simulink model "impendent_control"  (R2020b)
settings: Solver=FixedStepAuto  StartTime=0  StopTime=20  FixedStep=0.002  RelTol=1e-3
settings Model: Creator=lsk  LastModifiedBy=lsk

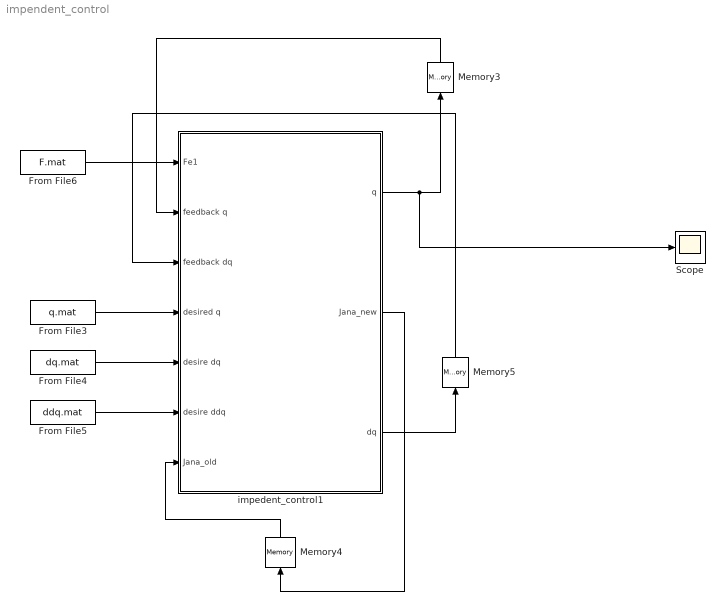
== system impendent_control ==
  From File3 : FromFile  FileName=q.mat
  From File4 : FromFile  FileName=dq.mat
  From File5 : FromFile  FileName=ddq.mat
  From File6 : FromFile  FileName=F.mat
  Memory3 : Memory  InitialCondition="[-1.26423369443190\t-1.44424631137251\t1.62606583856285\t-1.18060848187035\t-1.67197070062840\t-1.04318229967319]"
  Memory4 : Memory  InitialCondition="[-0.266147571210034\t-0.0228642277800098\t0.0561694595006700\t0.0432367769486852\t-0.0908701336324438\t0;-0.185625730629766\t0.0722313558368560\t-0.177447331936746\t-0.136591143644473\t-0.0343556248257271\t0;0\t-0.309757599949874\t-0.276437498712455\t-0.0433441320109634\t-0.00828008794975587\t0;0\t-0.611286356998400\t-0.611286356998400\t-0.611286356998400\t0.773691656626561\t-0.433817753420009;0\t0.832951080784977\t0.832951080784977\t0.832951080784977\t0.465262723808915\t-0.382135972757221;1\t-0.259766266542128\t-0.259766266542128\t-0.259766266542128\t-0.212540535977552\t-1.02086724969865]"
  Memory5 : Memory  InitialCondition="[0.0749188626195236\t0.110703858237117\t-0.193787178596464\t0.0894245369746680\t0.0405634935859376\t0.0633059717930151]"
  Scope : Scope
  impedent_control1 : Subsystem  mask{m_M=[1 1 1 1 1 1]*0.2, m_B=[1 1 1 1 1 1]*5, m_K=[1 1 1 1 1 1]*3}
      mask prompts: m_M "M"; m_B "B"; m_K "K"
  wires:
  From File6/1 -> impedent_control1/1(Fe1)
  From File4/1 -> impedent_control1/5(desire dq)
  impedent_control1/3(dq) -> Memory5/1
  Memory5/1 -> impedent_control1/3(feedback dq)
  impedent_control1/1(q) -> Scope/1, Memory3/1
  Memory3/1 -> impedent_control1/2(feedback q)
  Memory4/1 -> impedent_control1/7("Jana_old ")
  From File5/1 -> impedent_control1/6(desire ddq)
  impedent_control1/2(Jana_new) -> Memory4/1
  From File3/1 -> impedent_control1/4(desired q)

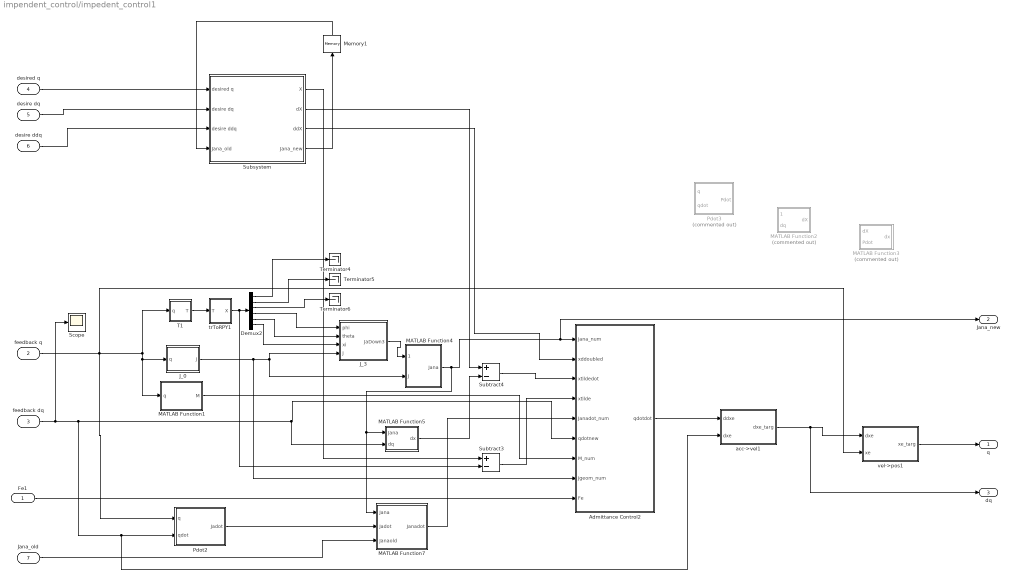
== system impendent_control/impedent_control1 ==
  Fe1 : Inport
  feedback q : Inport  Port=2
  feedback dq : Inport  Port=3
  desired q : Inport  Port=4
  desire dq : Inport  Port=5
  desire ddq : Inport  Port=6
  "Jana_old " : Inport  Port=7
  Admittance Control2 : MATLAB Function  TreatAsAtomicUnit=on
  Demux2 : Demux  Outputs=6
  J_0 : MATLAB Function  TreatAsAtomicUnit=on
  J_3 : MATLAB Function  TreatAsAtomicUnit=on
  MATLAB Function1 : MATLAB Function  TreatAsAtomicUnit=on
  MATLAB Function2 : MATLAB Function  Commented=on  TreatAsAtomicUnit=on
  MATLAB Function3 : MATLAB Function  Commented=on  TreatAsAtomicUnit=on
  MATLAB Function4 : MATLAB Function  TreatAsAtomicUnit=on
  MATLAB Function5 : MATLAB Function  TreatAsAtomicUnit=on
  MATLAB Function7 : MATLAB Function  TreatAsAtomicUnit=on
  Memory1 : Memory  InitialCondition="[-0.266147571210034\t-0.0228642277800098\t0.0561694595006700\t0.0432367769486852\t-0.0908701336324438\t0;-0.185625730629766\t0.0722313558368560\t-0.177447331936746\t-0.136591143644473\t-0.0343556248257271\t0;0\t-0.309757599949874\t-0.276437498712455\t-0.0433441320109634\t-0.00828008794975587\t0;0\t-0.611286356998400\t-0.611286356998400\t-0.611286356998400\t0.773691656626561\t-0.433817753420009;0\t0.832951080784977\t0.832951080784977\t0.832951080784977\t0.465262723808915\t-0.382135972757221;1\t-0.259766266542128\t-0.259766266542128\t-0.259766266542128\t-0.212540535977552\t-1.02086724969865]"
  Pdot2 : MATLAB Function  TreatAsAtomicUnit=on
  Pdot3 : MATLAB Function  Commented=on  TreatAsAtomicUnit=on
  Scope : Scope
  Subsystem : Subsystem
  Subtract3 : Sum  Inputs=+-
  Subtract4 : Sum  Inputs=+-
  T1 : MATLAB Function  TreatAsAtomicUnit=on
  Terminator4 : Terminator
  Terminator5 : Terminator
  Terminator6 : Terminator
  acc->vel1 : MATLAB Function  TreatAsAtomicUnit=on
  trToRPY1 : MATLAB Function  TreatAsAtomicUnit=on
  vel->pos1 : MATLAB Function  TreatAsAtomicUnit=on
  q : Outport
  Jana_new : Outport  Port=2
  dq : Outport  Port=3
  wires:
  acc->vel1/1(dxe_targ) -> dq/1, vel->pos1/1(dxe)
  T1/1(T) -> trToRPY1/1(T)
  trToRPY1/1(X) -> Subtract3/2, Demux2/1
  Demux2/3 -> Terminator6/1
  Demux2/2 -> Terminator5/1
  Demux2/1 -> Terminator4/1
  vel->pos1/1(xe_targ) -> q/1
  desired q/1 -> Subsystem/1(desired q)
  desire dq/1 -> Subsystem/2(desire dq)
  desire ddq/1 -> Subsystem/3(desire ddq)
  Subsystem/4(Jana_new) -> Memory1/1
  Memory1/1 -> Subsystem/4(Jana_old)
  feedback q/1 -> vel->pos1/2(xe), Pdot2/1(q), J_0/1(q), MATLAB Function1/1(q), T1/1(q)
  Demux2/4 -> J_3/1(phi)
  Demux2/5 -> J_3/2(theta)
  Demux2/6 -> J_3/3(xi)
  J_0/1(J) -> Admittance Control2/8(Jgeom_num), MATLAB Function4/2(J), J_3/4(J)
  J_3/1(JaDown3) -> MATLAB Function4/1(JaDown3)
  Subsystem/3(ddX) -> Admittance Control2/2(xddoubled)
  MATLAB Function4/1(Jana) -> MATLAB Function5/1(Jana), MATLAB Function7/1(Jana), Jana_new/1, Admittance Control2/1(Jana_num)
  feedback dq/1 -> acc->vel1/2(dxe), Pdot2/2(qdot), MATLAB Function5/2(dq), Admittance Control2/6(qdotnew), Scope/1
  Subsystem/2(dX) -> Subtract4/1
  MATLAB Function1/1(M) -> Admittance Control2/7(M_num)
  MATLAB Function5/1(dx) -> Subtract4/2
  Subtract4/1 -> Admittance Control2/3(xtildedot)
  Subsystem/1(X) -> Subtract3/1
  Subtract3/1 -> Admittance Control2/4(xtilde)
  Fe1/1 -> Admittance Control2/9(Fe)
  "Jana_old "/1 -> MATLAB Function7/3(Janaold)
  Pdot2/1(Jadot) -> MATLAB Function7/2(Jadot)
  MATLAB Function7/1(Janadot) -> Admittance Control2/5(Janadot_num)
  Admittance Control2/1(qdotdot) -> acc->vel1/1(ddxe)

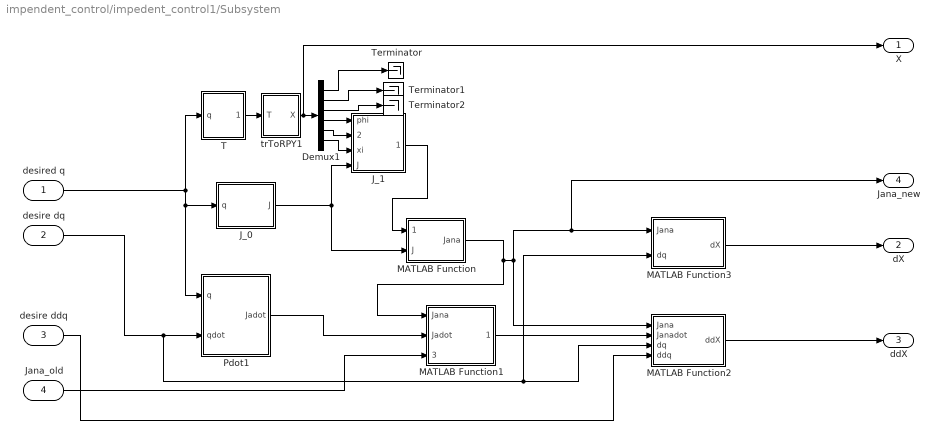
== system impendent_control/impedent_control1/Subsystem ==
  desired q : Inport
  desire dq : Inport  Port=2
  desire ddq : Inport  Port=3
  Jana_old : Inport  Port=4
  Demux1 : Demux  Outputs=6
  J_0 : MATLAB Function  TreatAsAtomicUnit=on
  J_1 : MATLAB Function  TreatAsAtomicUnit=on
  MATLAB Function : MATLAB Function  TreatAsAtomicUnit=on
  MATLAB Function1 : MATLAB Function  TreatAsAtomicUnit=on
  MATLAB Function2 : MATLAB Function  TreatAsAtomicUnit=on
  MATLAB Function3 : MATLAB Function  TreatAsAtomicUnit=on
  Pdot1 : MATLAB Function  TreatAsAtomicUnit=on
  T : MATLAB Function  TreatAsAtomicUnit=on
  Terminator : Terminator
  Terminator1 : Terminator
  Terminator2 : Terminator
  trToRPY1 : MATLAB Function  TreatAsAtomicUnit=on
  X : Outport
  dX : Outport  Port=2
  ddX : Outport  Port=3
  Jana_new : Outport  Port=4
  wires:
  desired q/1 -> Pdot1/1(q), J_0/1(q), T/1(q)
  T/1(T_fin) -> trToRPY1/1(T)
  Demux1/1 -> Terminator/1
  Demux1/2 -> Terminator1/1
  Demux1/6 -> J_1/3(xi)
  Demux1/3 -> Terminator2/1
  Demux1/4 -> J_1/1(phi)
  Demux1/5 -> J_1/2(theta)
  trToRPY1/1(X) -> X/1, Demux1/1
  J_0/1(J) -> MATLAB Function/2(J), J_1/4(J)
  J_1/1(JaDown3) -> MATLAB Function/1(JaDown3)
  desire dq/1 -> MATLAB Function2/3(dq), MATLAB Function3/2(dq), Pdot1/2(qdot)
  MATLAB Function/1(Jana) -> MATLAB Function1/1(Jana), MATLAB Function2/1(Jana), Jana_new/1, MATLAB Function3/1(Jana)
  Pdot1/1(Jadot) -> MATLAB Function1/2(Jadot)
  Jana_old/1 -> MATLAB Function1/3(Janaold)
  MATLAB Function3/1(dX) -> dX/1
  MATLAB Function1/1(Janadot) -> MATLAB Function2/2(Janadot)
  desire ddq/1 -> MATLAB Function2/4(ddq)
  MATLAB Function2/1(ddX) -> ddX/1

== matlab function impendent_control/impedent_control1/MATLAB Function7 ==
  data: Jana input; Jadot input; Janadot output; Janaold input
function Janadot = fcn(Jana,Jadot,Janaold)
Jadown3 = Jana - Janaold;
Janadot=[Jadot(1:3,:);Jadown3(4:6,:)];
end

== matlab function impendent_control/impedent_control1/Pdot2 ==
  data: q input; qdot input; Jadot output
function Jadot = Jadot(q,qdot)
%JADOT
%    JADOT = JADOT(Q1,Q2,Q3,Q4,Q5,Q1DOT,Q2DOT,Q3DOT,Q4DOT,Q5DOT)

%    This function was generated by the Symbolic Math Toolbox version 8.6.
%    07-Dec-2021 14:58:16
q1=q(1);q2=q(2);q3=q(3);q4=q(4);q5=q(5);q6=q(6);
q1dot=qdot(1);q2dot=qdot(2);q3dot=qdot(3);q4dot=qdot(4);q5dot=qdot(5);q6dot=qdot(6);
t2 = cos(q1);
t3 = cos(q2);
t4 = cos(q3);
t5 = cos(q4);
t6 = cos(q5);
t7 = sin(q1);
t8 = sin(q2);
t9 = sin(q3);
t10 = sin(q4);
t11 = sin(q5);
t12 = q2+q3+q4;
t13 = q2dot+q3dot+q4dot;
t14 = cos(t12);
t15 = sin(t12);
t16 = t6.*(3.9e+1./4.0e+2);
t17 = t5.*(5.7e+1./5.0e+2);
t18 = t10.*(5.7e+1./5.0e+2);
t22 = t5.*t11.*(3.9e+1./4.0e+2);
t23 = t10.*t11.*(3.9e+1./4.0e+2);
t24 = q4dot.*t10.*(-5.7e+1./5.0e+2);
t30 = q5dot.*t5.*t6.*(-3.9e+1./4.0e+2);
t19 = -t18;
t20 = q4dot.*t17;
t21 = q4dot.*t18;
t25 = -t22;
t26 = q5dot.*t5.*t16;
t27 = q4dot.*t22;
t28 = q5dot.*t10.*t16;
t29 = q4dot.*t23;
t31 = t16+1.065e-1;
t32 = t17+t23;
t33 = t18+t25;
t34 = t4.*t32;
t35 = t9.*t32;
t46 = t19+t22+2.37e+2./1.0e+3;
t51 = t20+t29+t30;
t52 = t24+t27+t28;
t36 = q3dot.*t34;
t37 = q3dot.*t35;
t38 = t4.*t33;
t39 = t9.*t33;
t42 = -t35;
t47 = t4.*t46;
t48 = t9.*t46;
t53 = t4.*t51;
t54 = t4.*t52;
t55 = t9.*t51;
t56 = t9.*t52;
t40 = q3dot.*t38;
t41 = q3dot.*t39;
t43 = -t37;
t44 = -t39;
t49 = q3dot.*t47;
t50 = q3dot.*t48;
t57 = -t54;
t58 = -t55;
t59 = t35+t38;
t66 = t34+t48;
t67 = t42+t47;
t72 = -t8.*(t35-t47);
t75 = -q2dot.*t3.*(t35-t47);
t45 = -t41;
t60 = t34+t44;
t61 = t8.*t59;
t62 = q2dot.*t3.*t59;
t68 = t3.*t66;
t69 = t8.*t66;
t76 = t67+3.3e+1./1.25e+2;
t85 = t37+t40+t55+t57;
t89 = t36+t50+t53+t56;
t92 = t43+t49+t54+t58;
t94 = -t3.*(t37-t49+t55+t57);
t95 = -t8.*(t37-t49+t55+t57);
t63 = t3.*t60;
t64 = -t61;
t65 = q2dot.*t8.*t60;
t70 = q2dot.*t69;
t71 = q2dot.*t68;
t73 = -t69;
t77 = t3.*t76;
t78 = t8.*t76;
t82 = t68+t72;
t84 = t36+t45+t53+t56;
t87 = t3.*t85;
t90 = t3.*t89;
t91 = t8.*t89;
t74 = -t70;
t79 = q2dot.*t78;
t80 = q2dot.*t77;
t81 = t63+t64;
t83 = t68+t78;
t86 = t73+t77;
t88 = t8.*t84;
t93 = -t91;
t96 = t62+t65+t87+t88;
t97 = t74+t75+t93+t94;
t98 = t71+t79+t90+t95;
t99 = t74+t80+t93+t94;
Jadot = reshape([-t7.*t98-q5dot.*t2.*t11.*(3.9e+1./4.0e+2)-q1dot.*t7.*t31-q1dot.*t2.*(t69-t77),t2.*t98-q5dot.*t7.*t11.*(3.9e+1./4.0e+2)+q1dot.*t2.*t31-q1dot.*t7.*(t69-t77),0.0,-t2.*(t70-t80+t91+t3.*(t37-t49+t55+t57))-q1dot.*t7.*t83,-t7.*(t70-t80+t91+t3.*(t37-t49+t55+t57))+q1dot.*t2.*t83,t98,-t2.*(t70+t91+t3.*(t37-t49+t55+t57)+q2dot.*t3.*(t35-t47))-q1dot.*t7.*t82,-t7.*(t70+t91+t3.*(t37-t49+t55+t57)+q2dot.*t3.*(t35-t47))+q1dot.*t2.*t82,t71+t90+t95+q2dot.*t72,-t2.*t96+q1dot.*t7.*(t61-t63),-t7.*t96-q1dot.*t2.*(t61-t63),q2dot.*t63+q2dot.*t64+t3.*t84-t8.*t85,q1dot.*t2.*t11.*(-3.9e+1./4.0e+2)-q5dot.*t6.*t7.*(3.9e+1./4.0e+2)+q5dot.*t2.*t11.*t14.*(3.9e+1./4.0e+2)+q1dot.*t7.*t14.*t16+t2.*t13.*t15.*t16,q1dot.*t7.*t11.*(-3.9e+1./4.0e+2)+q5dot.*t2.*t16-q1dot.*t2.*t6.*t14.*(3.9e+1./4.0e+2)+q5dot.*t7.*t11.*t14.*(3.9e+1./4.0e+2)+t7.*t13.*t15.*t16,q5dot.*t11.*t15.*(3.9e+1./4.0e+2)-t6.*t13.*t14.*(3.9e+1./4.0e+2),0.0,0.0,0.0],[3,6]);

end

== matlab function impendent_control/impedent_control1/Pdot3 ==
  data: q input; qdot input; Pdot output
% function Pdot = Pdot(q1,q2,q3,q4,q5,q1dot,q2dot,q3dot,q4dot,q5dot)
function Pdot = Pdot(q,qdot)
q1=q(1);q2=q(2);q3=q(3);q4=q(4);q5=q(5);q6=q(6);
q1dot=qdot(1);q2dot=qdot(2);q3dot=qdot(3);q4dot=qdot(4);q5dot=qdot(5);q6dot=qdot(6);
%PDOT
%    PDOT = PDOT(Q1,Q2,Q3,Q4,Q5,Q1DOT,Q2DOT,Q3DOT,Q4DOT,Q5DOT)

%    This function was generated by the Symbolic Math Toolbox version 8.6.
%    07-Dec-2021 16:11:39

t2 = cos(q1);
t3 = cos(q2);
t4 = cos(q3);
t5 = cos(q4);
t6 = cos(q5);
t7 = sin(q1);
t8 = sin(q2);
t9 = sin(q3);
t10 = sin(q4);
t11 = sin(q5);
t12 = t6.*(3.9e+1./4.0e+2);
t13 = t5.*(5.7e+1./5.0e+2);
t14 = t10.*(5.7e+1./5.0e+2);
t18 = t5.*t11.*(3.9e+1./4.0e+2);
t19 = t10.*t11.*(3.9e+1./4.0e+2);
t20 = q4dot.*t10.*(-5.7e+1./5.0e+2);
t25 = q5dot.*t5.*t6.*(-3.9e+1./4.0e+2);
t15 = -t14;
t16 = q4dot.*t13;
t17 = q4dot.*t14;
t21 = q5dot.*t5.*t12;
t22 = q4dot.*t18;
t23 = q5dot.*t10.*t12;
t24 = q4dot.*t19;
t26 = t12+1.065e-1;
t27 = t13+t19;
t28 = t4.*t27;
t29 = t9.*t27;
t34 = t15+t18+2.37e+2./1.0e+3;
t39 = t16+t24+t25;
t40 = t20+t22+t23;
t30 = q3dot.*t28;
t31 = q3dot.*t29;
t32 = -t29;
t35 = t4.*t34;
t36 = t9.*t34;
t41 = t4.*t39;
t42 = t4.*t40;
t43 = t9.*t39;
t44 = t9.*t40;
t33 = -t31;
t37 = q3dot.*t35;
t38 = q3dot.*t36;
t45 = -t43;
t46 = t28+t36;
t50 = t32+t35+3.3e+1./1.25e+2;
t47 = t8.*t46;
t48 = q2dot.*t3.*t46;
t51 = t3.*t50;
t52 = q2dot.*t8.*t50;
t54 = t30+t38+t41+t44;
t56 = t33+t37+t42+t45;
t57 = -t8.*(t31-t37-t42+t43);
t49 = -t47;
t55 = t3.*t54;
t53 = t49+t51;
t58 = t48+t52+t55+t57;
Pdot = [t2.*t58-q5dot.*t7.*t11.*(3.9e+1./4.0e+2)+q1dot.*t2.*t26-q1dot.*t7.*(t47-t51);t7.*t58+q5dot.*t2.*t11.*(3.9e+1./4.0e+2)+q1dot.*t7.*t26+q1dot.*t2.*(t47-t51);q2dot.*t47-q2dot.*t51+t8.*t54+t3.*(t31-t37-t42+t43)];


end

== matlab function impendent_control/impedent_control1/Subsystem/J_0 ==
  data: q input; J output
function J = J(q)
q1=q(1);q2=q(2);q3=q(3);q4=q(4);q5=q(5);q6=q(6);
%J
%    J = J(Q1,Q2,Q3,Q4,Q5)

%    This function was generated by the Symbolic Math Toolbox version 8.6.
%    07-Dec-2021 11:30:25

t2 = cos(q1);
t3 = cos(q2);
t4 = cos(q3);
t5 = cos(q4);
t6 = cos(q5);
t7 = sin(q1);
t8 = sin(q2);
t9 = sin(q3);
t10 = sin(q4);
t11 = sin(q5);
t12 = q2+q3+q4;
t13 = cos(t12);
t14 = sin(t12);
t15 = -t2;
t16 = t6.*(3.9e+1./4.0e+2);
t17 = t5.*(5.7e+1./5.0e+2);
t18 = t10.*(5.7e+1./5.0e+2);
t20 = t5.*t11.*(3.9e+1./4.0e+2);
t21 = t10.*t11.*(3.9e+1./4.0e+2);
t19 = -t18;
t22 = -t20;
t23 = t16+1.065e-1;
t24 = t17+t21;
t25 = t18+t22;
t26 = t4.*t24;
t27 = t9.*t24;
t32 = t19+t20+2.37e+2./1.0e+3;
t28 = t4.*t25;
t29 = t9.*t25;
t30 = -t27;
t33 = t4.*t32;
t34 = t9.*t32;
t31 = -t29;
t35 = t27+t28;
t40 = t26+t34;
t41 = t30+t33;
t44 = -t8.*(t27-t33);
t36 = t26+t31;
t37 = t8.*t35;
t42 = t3.*t40;
t43 = t8.*t40;
t46 = t41+3.3e+1./1.25e+2;
t38 = t3.*t36;
t39 = -t37;
t45 = -t43;
t47 = t3.*t46;
t48 = t8.*t46;
t50 = t42+t44;
t49 = t38+t39;
t51 = t42+t48;
t52 = t45+t47;
J = reshape([t2.*t23-t7.*(t43-t47),t7.*t23+t2.*(t43-t47),0.0,0.0,0.0,1.0,t2.*t51,t7.*t51,t43-t47,t7,t15,0.0,t2.*t50,t7.*t50,t43+t3.*(t27-t33),t7,t15,0.0,-t2.*(t37-t38),-t7.*(t37-t38),t3.*t35+t8.*t36,t7,t15,0.0,t7.*t11.*(-3.9e+1./4.0e+2)-t2.*t6.*t13.*(3.9e+1./4.0e+2),t2.*t11.*(3.9e+1./4.0e+2)-t6.*t7.*t13.*(3.9e+1./4.0e+2),t6.*t14.*(-3.9e+1./4.0e+2),t2.*t14,t7.*t14,-t13,0.0,0.0,0.0,t6.*t7+t11.*t13.*t15,t6.*t15-t7.*t11.*t13,-t11.*t14],[6,6]);


end

== matlab function impendent_control/impedent_control1/Subsystem/J_1 ==
  data: phi input; JaDown3 output; theta input; xi input; J input
function JaDown3 = Jana(phi,theta,xi,J)
om2eulmat=[cos(theta)*cos(xi), -sin(xi), 0;
    cos(theta)*sin(xi),  cos(xi), 0;
    -sin(theta),       0, 1];
omega=J(4:6,:);
JaDown3 = om2eulmat\omega;
end

== matlab function impendent_control/impedent_control1/Subsystem/MATLAB Function ==
  data: JaDown3 input; Jana output; J input
function Jana = fcn(JaDown3,J)
Jana=[J(1:3,:);JaDown3];
end

== matlab function impendent_control/impedent_control1/Subsystem/MATLAB Function1 ==
  data: Jana input; Jadot input; Janadot output; Janaold input
function Janadot = fcn(Jana,Jadot,Janaold)
Jadown3 = Jana - Janaold;
Janadot=[Jadot(1:3,:);Jadown3(4:6,:)];
end

== matlab function impendent_control/impedent_control1/Subsystem/MATLAB Function2 ==
  data: Jana input; Janadot input; dq input; ddX output; ddq input
function ddX = getddX(Jana,Janadot,dq,ddq)
ddX = Janadot * dq + Jana * ddq;

== matlab function impendent_control/impedent_control1/Subsystem/MATLAB Function3 ==
  data: Jana input; dX output; dq input
function dX = getdX(Jana,dq)
dX=Jana*dq;

== matlab function impendent_control/impedent_control1/Subsystem/Pdot1 ==
  data: q input; qdot input; Jadot output
function Jadot = Jadot(q,qdot)
%JADOT
%    JADOT = JADOT(Q1,Q2,Q3,Q4,Q5,Q1DOT,Q2DOT,Q3DOT,Q4DOT,Q5DOT)

%    This function was generated by the Symbolic Math Toolbox version 8.6.
%    07-Dec-2021 14:58:16
q1=q(1);q2=q(2);q3=q(3);q4=q(4);q5=q(5);q6=q(6);
q1dot=qdot(1);q2dot=qdot(2);q3dot=qdot(3);q4dot=qdot(4);q5dot=qdot(5);q6dot=qdot(6);
t2 = cos(q1);
t3 = cos(q2);
t4 = cos(q3);
t5 = cos(q4);
t6 = cos(q5);
t7 = sin(q1);
t8 = sin(q2);
t9 = sin(q3);
t10 = sin(q4);
t11 = sin(q5);
t12 = q2+q3+q4;
t13 = q2dot+q3dot+q4dot;
t14 = cos(t12);
t15 = sin(t12);
t16 = t6.*(3.9e+1./4.0e+2);
t17 = t5.*(5.7e+1./5.0e+2);
t18 = t10.*(5.7e+1./5.0e+2);
t22 = t5.*t11.*(3.9e+1./4.0e+2);
t23 = t10.*t11.*(3.9e+1./4.0e+2);
t24 = q4dot.*t10.*(-5.7e+1./5.0e+2);
t30 = q5dot.*t5.*t6.*(-3.9e+1./4.0e+2);
t19 = -t18;
t20 = q4dot.*t17;
t21 = q4dot.*t18;
t25 = -t22;
t26 = q5dot.*t5.*t16;
t27 = q4dot.*t22;
t28 = q5dot.*t10.*t16;
t29 = q4dot.*t23;
t31 = t16+1.065e-1;
t32 = t17+t23;
t33 = t18+t25;
t34 = t4.*t32;
t35 = t9.*t32;
t46 = t19+t22+2.37e+2./1.0e+3;
t51 = t20+t29+t30;
t52 = t24+t27+t28;
t36 = q3dot.*t34;
t37 = q3dot.*t35;
t38 = t4.*t33;
t39 = t9.*t33;
t42 = -t35;
t47 = t4.*t46;
t48 = t9.*t46;
t53 = t4.*t51;
t54 = t4.*t52;
t55 = t9.*t51;
t56 = t9.*t52;
t40 = q3dot.*t38;
t41 = q3dot.*t39;
t43 = -t37;
t44 = -t39;
t49 = q3dot.*t47;
t50 = q3dot.*t48;
t57 = -t54;
t58 = -t55;
t59 = t35+t38;
t66 = t34+t48;
t67 = t42+t47;
t72 = -t8.*(t35-t47);
t75 = -q2dot.*t3.*(t35-t47);
t45 = -t41;
t60 = t34+t44;
t61 = t8.*t59;
t62 = q2dot.*t3.*t59;
t68 = t3.*t66;
t69 = t8.*t66;
t76 = t67+3.3e+1./1.25e+2;
t85 = t37+t40+t55+t57;
t89 = t36+t50+t53+t56;
t92 = t43+t49+t54+t58;
t94 = -t3.*(t37-t49+t55+t57);
t95 = -t8.*(t37-t49+t55+t57);
t63 = t3.*t60;
t64 = -t61;
t65 = q2dot.*t8.*t60;
t70 = q2dot.*t69;
t71 = q2dot.*t68;
t73 = -t69;
t77 = t3.*t76;
t78 = t8.*t76;
t82 = t68+t72;
t84 = t36+t45+t53+t56;
t87 = t3.*t85;
t90 = t3.*t89;
t91 = t8.*t89;
t74 = -t70;
t79 = q2dot.*t78;
t80 = q2dot.*t77;
t81 = t63+t64;
t83 = t68+t78;
t86 = t73+t77;
t88 = t8.*t84;
t93 = -t91;
t96 = t62+t65+t87+t88;
t97 = t74+t75+t93+t94;
t98 = t71+t79+t90+t95;
t99 = t74+t80+t93+t94;
Jadot = reshape([-t7.*t98-q5dot.*t2.*t11.*(3.9e+1./4.0e+2)-q1dot.*t7.*t31-q1dot.*t2.*(t69-t77),t2.*t98-q5dot.*t7.*t11.*(3.9e+1./4.0e+2)+q1dot.*t2.*t31-q1dot.*t7.*(t69-t77),0.0,-t2.*(t70-t80+t91+t3.*(t37-t49+t55+t57))-q1dot.*t7.*t83,-t7.*(t70-t80+t91+t3.*(t37-t49+t55+t57))+q1dot.*t2.*t83,t98,-t2.*(t70+t91+t3.*(t37-t49+t55+t57)+q2dot.*t3.*(t35-t47))-q1dot.*t7.*t82,-t7.*(t70+t91+t3.*(t37-t49+t55+t57)+q2dot.*t3.*(t35-t47))+q1dot.*t2.*t82,t71+t90+t95+q2dot.*t72,-t2.*t96+q1dot.*t7.*(t61-t63),-t7.*t96-q1dot.*t2.*(t61-t63),q2dot.*t63+q2dot.*t64+t3.*t84-t8.*t85,q1dot.*t2.*t11.*(-3.9e+1./4.0e+2)-q5dot.*t6.*t7.*(3.9e+1./4.0e+2)+q5dot.*t2.*t11.*t14.*(3.9e+1./4.0e+2)+q1dot.*t7.*t14.*t16+t2.*t13.*t15.*t16,q1dot.*t7.*t11.*(-3.9e+1./4.0e+2)+q5dot.*t2.*t16-q1dot.*t2.*t6.*t14.*(3.9e+1./4.0e+2)+q5dot.*t7.*t11.*t14.*(3.9e+1./4.0e+2)+t7.*t13.*t15.*t16,q5dot.*t11.*t15.*(3.9e+1./4.0e+2)-t6.*t13.*t14.*(3.9e+1./4.0e+2),0.0,0.0,0.0],[3,6]);

end

== matlab function impendent_control/impedent_control1/Subsystem/T ==
  data: q input; T_fin output
function T_fin = transion(q)
q1=q(1);q2=q(2);q3=q(3);q4=q(4);q5=q(5);q6=q(6);
t2 = cos(q1);
t3 = cos(q2);
t4 = cos(q3);
t5 = cos(q4);
t6 = cos(q5);
t7 = cos(q6);
t8 = sin(q1);
t9 = sin(q2);
t10 = sin(q3);
t11 = sin(q4);
t12 = sin(q5);
t13 = sin(q6);
t14 = q2+q3+q4;
t15 = cos(t14);
t16 = t2.*t12;
t17 = sin(t14);
t18 = t8.*t12;
t19 = t6.*(3.9e+1./4.0e+2);
t20 = t5.*(5.7e+1./5.0e+2);
t21 = t11.*(5.7e+1./5.0e+2);
t25 = t5.*t12.*(3.9e+1./4.0e+2);
t26 = t11.*t12.*(3.9e+1./4.0e+2);
t22 = t2.*t6.*t15;
t23 = t6.*t8.*t15;
t24 = -t21;
t29 = t19+1.065e-1;
t31 = t20+t26;
t27 = -t23;
t28 = t18+t22;
t32 = t4.*t31;
t33 = t10.*t31;
t35 = t24+t25+2.37e+2./1.0e+3;
t30 = t16+t27;
t34 = -t33;
t36 = t4.*t35;
t37 = t10.*t35;
t38 = t32+t37;
t41 = t34+t36+3.3e+1./1.25e+2;
t39 = t9.*t38;
t42 = t3.*t41;
t40 = -t39;
T_fin = reshape([t7.*t28-t2.*t13.*t17,-t7.*t30-t8.*t13.*t17,t13.*t15+t6.*t7.*t17,0.0,-t13.*t28-t2.*t7.*t17,t13.*t30-t7.*t8.*t17,t7.*t15-t6.*t13.*t17,0.0,t6.*t8-t15.*t16,-t2.*t6-t15.*t18,-t12.*t17,0.0,t8.*t29+t2.*(t39-t42),-t2.*t29+t8.*(t39-t42),-t3.*t38-t9.*t41+1.8e+1./1.25e+2,1.0],[4,4]);
end

== matlab function impendent_control/impedent_control1/Subsystem/trToRPY1 ==
  data: T input; X output
function  X=Tr2Pos(T)
%#codegen
coder.extrinsic('disp'); %Declare disp as extrinsic
    %% 求末端位置
    x=T(1,4);y=T(2,4);z=T(3,4);
    %% 根据X-Y-Z固定角计算
    R=T;rpy=[0,0,0];
    if abs(abs(R(3,1)) - 1) < 0.000001  % when |R31| == 1
    % singularity
        rpy(1) = 0;     % roll is zero
        if R(3,1) < 0
            rpy(3) = -atan2(R(1,2), R(1,3));  % R-Y
        else
            rpy(3) = atan2(-R(1,2), -R(1,3));  % R+Y
        end
        rpy(2) = -asin(R(3,1));
    else
        rpy(1) = atan2(R(3,2), R(3,3));  % R
        rpy(3) = atan2(R(2,1), R(1,1));  % Y

        [~,k] = max(abs( [R(1,1) R(2,1) R(3,2) R(3,3)] ));
        switch k
            case 1
                rpy(2) = -atan(R(3,1)*cos(rpy(3))/R(1,1));
            case 2
                rpy(2) = -atan(R(3,1)*sin(rpy(3))/R(2,1));
            case 3
                rpy(2) = -atan(R(3,1)*sin(rpy(1))/R(3,2));
            case 4
                rpy(2) = -atan(R(3,1)*cos(rpy(1))/R(3,3));
        end
    end
%     RPY=rpy*180/pi;
    RPY=rpy;
    Roll=RPY(1);Pitch=RPY(2);Yaw=RPY(3);
    X=[x,y,z,Roll,Pitch,Yaw];
end

== matlab function impendent_control/impedent_control1/T1 ==
  data: q input; T output
function T = transion(q)
q1=q(1);q2=q(2);q3=q(3);q4=q(4);q5=q(5);q6=q(6);
t2 = cos(q1);
t3 = cos(q2);
t4 = cos(q3);
t5 = cos(q4);
t6 = cos(q5);
t7 = cos(q6);
t8 = sin(q1);
t9 = sin(q2);
t10 = sin(q3);
t11 = sin(q4);
t12 = sin(q5);
t13 = sin(q6);
t14 = q2+q3+q4;
t15 = cos(t14);
t16 = t2.*t12;
t17 = sin(t14);
t18 = t8.*t12;
t19 = t6.*(3.9e+1./4.0e+2);
t20 = t5.*(5.7e+1./5.0e+2);
t21 = t11.*(5.7e+1./5.0e+2);
t25 = t5.*t12.*(3.9e+1./4.0e+2);
t26 = t11.*t12.*(3.9e+1./4.0e+2);
t22 = t2.*t6.*t15;
t23 = t6.*t8.*t15;
t24 = -t21;
t29 = t19+1.065e-1;
t31 = t20+t26;
t27 = -t23;
t28 = t18+t22;
t32 = t4.*t31;
t33 = t10.*t31;
t35 = t24+t25+2.37e+2./1.0e+3;
t30 = t16+t27;
t34 = -t33;
t36 = t4.*t35;
t37 = t10.*t35;
t38 = t32+t37;
t41 = t34+t36+3.3e+1./1.25e+2;
t39 = t9.*t38;
t42 = t3.*t41;
t40 = -t39;
T = reshape([t7.*t28-t2.*t13.*t17,-t7.*t30-t8.*t13.*t17,t13.*t15+t6.*t7.*t17,0.0,-t13.*t28-t2.*t7.*t17,t13.*t30-t7.*t8.*t17,t7.*t15-t6.*t13.*t17,0.0,t6.*t8-t15.*t16,-t2.*t6-t15.*t18,-t12.*t17,0.0,t8.*t29+t2.*(t39-t42),-t2.*t29+t8.*(t39-t42),-t3.*t38-t9.*t41+1.8e+1./1.25e+2,1.0],[4,4]);
end

== matlab function impendent_control/impedent_control1/acc->vel1 ==
  data: ddxe input; dxe input; dxe_targ output
function dxe_targ   = acc_integral(ddxe,dxe)
%% parameter
% dt = 0.001;
dt = 0.02;
dxe_targ=zeros(1,6);
dt_ddxe=ddxe*dt;
dxe_targ(1)=dxe(1)+dt_ddxe(1);
dxe_targ(2)=dxe(2)+dt_ddxe(2);
dxe_targ(3)=dxe(3)+dt_ddxe(3);
dxe_targ(4)=dxe(4)+dt_ddxe(4);
dxe_targ(5)=dxe(5)+dt_ddxe(5);
dxe_targ(6)=dxe(6)+dt_ddxe(6);
end

== matlab function impendent_control/impedent_control1/trToRPY1 ==
  data: T input; X output
function  X=Tr2Pos(T)
%#codegen
coder.extrinsic('disp'); %Declare disp as extrinsic
    %% 求末端位置
    x=T(1,4);y=T(2,4);z=T(3,4);
    %% 根据X-Y-Z固定角计算
    R=T;rpy=[0,0,0];
    if abs(abs(R(3,1)) - 1) < 0.000001  % when |R31| == 1
    % singularity
        rpy(1) = 0;     % roll is zero
        if R(3,1) < 0
            rpy(3) = -atan2(R(1,2), R(1,3));  % R-Y
        else
            rpy(3) = atan2(-R(1,2), -R(1,3));  % R+Y
        end
        rpy(2) = -asin(R(3,1));
    else
        rpy(1) = atan2(R(3,2), R(3,3));  % R
        rpy(3) = atan2(R(2,1), R(1,1));  % Y

        [~,k] = max(abs( [R(1,1) R(2,1) R(3,2) R(3,3)] ));
        switch k
            case 1
                rpy(2) = -atan(R(3,1)*cos(rpy(3))/R(1,1));
            case 2
                rpy(2) = -atan(R(3,1)*sin(rpy(3))/R(2,1));
            case 3
                rpy(2) = -atan(R(3,1)*sin(rpy(1))/R(3,2));
            case 4
                rpy(2) = -atan(R(3,1)*cos(rpy(1))/R(3,3));
        end
    end
%     RPY=rpy*180/pi;
    RPY=rpy;
    Roll=RPY(1);Pitch=RPY(2);Yaw=RPY(3);
    X=[x,y,z,Roll,Pitch,Yaw];
end

== matlab function impendent_control/impedent_control1/vel->pos1 ==
  data: dxe input; xe input; xe_targ output
function xe_targ   = vel_integral(dxe,xe)
%% parameter
xe_targ=zeros(1,6);
% dt = 0.001;
dt = 0.02;
dt_dxe=dxe*dt;
xe_targ(1)=xe(1)+dt_dxe(1);
xe_targ(2)=xe(2)+dt_dxe(2);
xe_targ(3)=xe(3)+dt_dxe(3);
xe_targ(4)=xe(4)+dt_dxe(4);
xe_targ(5)=xe(5)+dt_dxe(5);
xe_targ(6)=xe(6)+dt_dxe(6);

end

== matlab function impendent_control/impedent_control1/Admittance Control2 ==
  data: Jana_num input; xddoubled input; m_M parameter; m_B parameter; m_K parameter; xtildedot input; xtilde input; Janadot_num input; qdotnew input; M_num input; Jgeom_num input; qdotdot output; Fe input
function qdotdot  = fcn(Jana_num, xddoubled ,m_M, m_B, m_K, xtildedot ,xtilde ,Janadot_num ,qdotnew ,M_num ,Jgeom_num, Fe)

%% control parameter
qdotdot=zeros(6,1);
Md = diag(m_M);
Kd = diag(m_B);
Kp = diag(m_K);

% qdotdot = Jana_num\(xddoubled + Md\Kd*xtildedot + Md\Kp*xtilde' - Janadot_num*qdotnew) - M_num\Jgeom_num'*Fe;
qdotdot = Jana_num\(xddoubled + Md\Kd*xtildedot + Md\Kp*xtilde' - Janadot_num*qdotnew) - eye(6)\Jgeom_num'*Fe;

end

== matlab function impendent_control/impedent_control1/J_0 ==
  data: q input; J output
function J = J(q)
q1=q(1);q2=q(2);q3=q(3);q4=q(4);q5=q(5);q6=q(6);
%J
%    J = J(Q1,Q2,Q3,Q4,Q5)

%    This function was generated by the Symbolic Math Toolbox version 8.6.
%    07-Dec-2021 11:30:25

t2 = cos(q1);
t3 = cos(q2);
t4 = cos(q3);
t5 = cos(q4);
t6 = cos(q5);
t7 = sin(q1);
t8 = sin(q2);
t9 = sin(q3);
t10 = sin(q4);
t11 = sin(q5);
t12 = q2+q3+q4;
t13 = cos(t12);
t14 = sin(t12);
t15 = -t2;
t16 = t6.*(3.9e+1./4.0e+2);
t17 = t5.*(5.7e+1./5.0e+2);
t18 = t10.*(5.7e+1./5.0e+2);
t20 = t5.*t11.*(3.9e+1./4.0e+2);
t21 = t10.*t11.*(3.9e+1./4.0e+2);
t19 = -t18;
t22 = -t20;
t23 = t16+1.065e-1;
t24 = t17+t21;
t25 = t18+t22;
t26 = t4.*t24;
t27 = t9.*t24;
t32 = t19+t20+2.37e+2./1.0e+3;
t28 = t4.*t25;
t29 = t9.*t25;
t30 = -t27;
t33 = t4.*t32;
t34 = t9.*t32;
t31 = -t29;
t35 = t27+t28;
t40 = t26+t34;
t41 = t30+t33;
t44 = -t8.*(t27-t33);
t36 = t26+t31;
t37 = t8.*t35;
t42 = t3.*t40;
t43 = t8.*t40;
t46 = t41+3.3e+1./1.25e+2;
t38 = t3.*t36;
t39 = -t37;
t45 = -t43;
t47 = t3.*t46;
t48 = t8.*t46;
t50 = t42+t44;
t49 = t38+t39;
t51 = t42+t48;
t52 = t45+t47;
J = reshape([t2.*t23-t7.*(t43-t47),t7.*t23+t2.*(t43-t47),0.0,0.0,0.0,1.0,t2.*t51,t7.*t51,t43-t47,t7,t15,0.0,t2.*t50,t7.*t50,t43+t3.*(t27-t33),t7,t15,0.0,-t2.*(t37-t38),-t7.*(t37-t38),t3.*t35+t8.*t36,t7,t15,0.0,t7.*t11.*(-3.9e+1./4.0e+2)-t2.*t6.*t13.*(3.9e+1./4.0e+2),t2.*t11.*(3.9e+1./4.0e+2)-t6.*t7.*t13.*(3.9e+1./4.0e+2),t6.*t14.*(-3.9e+1./4.0e+2),t2.*t14,t7.*t14,-t13,0.0,0.0,0.0,t6.*t7+t11.*t13.*t15,t6.*t15-t7.*t11.*t13,-t11.*t14],[6,6]);


end

== matlab function impendent_control/impedent_control1/J_3 ==
  data: phi input; JaDown3 output; theta input; xi input; J input
function JaDown3 = Jana(phi,theta,xi,J)
om2eulmat=[cos(theta)*cos(xi), -sin(xi), 0;
    cos(theta)*sin(xi),  cos(xi), 0;
    -sin(theta),       0, 1];
omega=J(4:6,:);
JaDown3 = om2eulmat\omega;
end

== matlab function impendent_control/impedent_control1/MATLAB Function1 ==
  data: q input; M output
function M = M_num(q)
%M_NUM
%    M = M_NUM(Q1,Q2,Q3,Q4,Q5,Q6)
q1=q(1);q2=q(2);q3=q(3);q4=q(4);q5=q(5);q6=q(6);
%    This function was generated by the Symbolic Math Toolbox version 8.6.
%    07-Dec-2021 16:24:19

t2 = cos(q1);
t3 = cos(q2);
t4 = cos(q3);
t5 = cos(q4);
t6 = cos(q5);
t7 = cos(q6);
t8 = sin(q1);
t9 = sin(q2);
t10 = sin(q3);
t11 = sin(q4);
t12 = sin(q5);
t13 = sin(q6);
t14 = q2+q3;
t15 = q2+q5;
t16 = q3+q4;
t17 = q2.*2.0;
t18 = q3.*2.0;
t19 = q4.*2.0;
t20 = q5.*2.0;
t21 = q6.*2.0;
t33 = -q5;
t22 = t6.^2;
t23 = t7.^2;
t24 = sin(t20);
t25 = cos(t14);
t26 = cos(t15);
t27 = cos(t16);
t28 = q4+t14;
t29 = q5+t14;
t30 = sin(t14);
t31 = sin(t15);
t32 = sin(t16);
t34 = -t20;
t35 = -t21;
t36 = t2.*t6;
t39 = t2.*t12;
t40 = t6.*t8;
t44 = t8.*t12;
t45 = q2+t14;
t49 = q2+t33;
t50 = t14.*2.0;
t52 = t14+t33;
t64 = t6.*(3.9e+1./4.0e+2);
t65 = t5.*(5.7e+1./5.0e+2);
t66 = t11.*(5.7e+1./5.0e+2);
t83 = t5.*t12.*(3.9e+1./4.0e+2);
t84 = t11.*t12.*(3.9e+1./4.0e+2);
t99 = t4.*1.014787488e-1;
t121 = t6.*2.10083e-2;
t122 = t12.*2.10083e-2;
t125 = t6.*1.5925e-4;
t127 = t6.*8.86e-5;
t128 = t12.*8.86e-5;
t129 = t7.*t12.*t13.*1.889999999999997e-6;
t132 = t11.*1.114986e-1;
t136 = t5.*1.114986e-1;
t140 = t10.*2.65188e-5;
t146 = t5.*7.16878548e-5;
t152 = t5.*3.58439274e-5;
t163 = t11.*t12.*3.58439274e-5;
t164 = t4.*t5.*t6.*3.99274128e-5;
t165 = t4.*t11.*t12.*3.99274128e-5;
t166 = t5.*t10.*t12.*3.99274128e-5;
t167 = t6.*t10.*t11.*3.99274128e-5;
t169 = t5.*t12.*4.4321768397e-3;
t170 = t5.*t12.*8.8643536794e-3;
t171 = t6.*t11.*4.4321768397e-3;
t176 = t4.*t5.*t12.*4.9371083784e-3;
t177 = t4.*t6.*t11.*4.9371083784e-3;
t178 = t5.*t6.*t10.*4.9371083784e-3;
t179 = t10.*t11.*t12.*4.9371083784e-3;
t184 = t11.*8.27276665554e-2;
t197 = t11.*4.13638332777e-2;
t202 = t4.*t11.*5.55435170928e-2;
t203 = t5.*t10.*5.55435170928e-2;
t222 = t3.*1.5989248968e-5;
t225 = t9.*5.962436486703985e-3;
t230 = t12.*9.06307056372e-6;
t234 = t6.*1.94303003751466e-3;
t37 = cos(t28);
t38 = cos(t29);
t41 = q5+t28;
t42 = sin(t28);
t43 = sin(t29);
t46 = q2+t28;
t51 = cos(t49);
t53 = sin(t49);
t54 = t20+t28;
t57 = t14+t28;
t58 = cos(t52);
t59 = t28+t33;
t60 = t28+t34;
t61 = sin(t52);
t80 = -t66;
t82 = t19+t50;
t85 = -t83;
t93 = t64+1.065e-1;
t100 = t65+t84;
t123 = -t122;
t124 = t23.*1.889999999999997e-6;
t137 = -t132;
t147 = t31.*4.7336741892e-3;
t148 = t32.*9.4673483784e-3;
t149 = t26.*1.99637064e-5;
t150 = t27.*3.99274128e-5;
t151 = -t146;
t157 = t6.*t146;
t158 = -t152;
t161 = t6.*t152;
t175 = -t163;
t180 = -t165;
t181 = -t166;
t182 = -t167;
t185 = -t170;
t186 = -t169;
t187 = -t171;
t190 = t25.*1.6725731e-5;
t192 = -t176;
t193 = -t177;
t194 = -t178;
t196 = -t184;
t200 = -t197;
t206 = -t202;
t207 = -t203;
t214 = t30.*7.78686501734e-2;
t223 = t24.*9.27729949366e-6;
t240 = t121+t128-1.065e-1;
t252 = t22.*2.77326877791351e-3;
t277 = t129+t230+t234;
t47 = cos(t41);
t48 = sin(t41);
t55 = t7.*t37;
t56 = t13.*t37;
t62 = cos(t54);
t63 = sin(t54);
t67 = cos(t59);
t68 = cos(t60);
t69 = sin(t59);
t70 = sin(t60);
t71 = t36.*t37;
t72 = t37.*t39;
t73 = t37.*t40;
t74 = t2.*t7.*t42;
t75 = t6.*t7.*t42;
t76 = t37.*t44;
t77 = t2.*t13.*t42;
t78 = t7.*t8.*t42;
t79 = t6.*t13.*t42;
t81 = t8.*t13.*t42;
t101 = t2.*t93;
t102 = t8.*t93;
t106 = t66+t85;
t108 = t4.*t100;
t109 = t10.*t100;
t115 = t80+t83+2.37e+2./1.0e+3;
t126 = -t124;
t131 = t22.*t124;
t141 = t24.*t42.*7.962500000000001e-5;
t153 = -t147;
t154 = -t149;
t155 = -t150;
t159 = t53.*4.7336741892e-3;
t162 = t43.*4.24954841985e-3;
t168 = t38.*1.79219637e-5;
t173 = t51.*1.99637064e-5;
t195 = t61.*4.24954841985e-3;
t198 = -t190;
t201 = t58.*1.79219637e-5;
t224 = t123+t127;
t226 = -t223;
t238 = t42.*7.92876906372e-6;
t245 = t37.*1.663963245953534e-2;
t255 = -t252;
t298 = t175+t187+t277;
t86 = -t72;
t87 = -t73;
t88 = -t77;
t89 = -t78;
t90 = -t79;
t91 = t36+t76;
t92 = t44+t71;
t97 = t56+t75;
t107 = -t102;
t110 = t4.*t106;
t111 = t10.*t106;
t112 = -t109;
t118 = t4.*t115;
t119 = t10.*t115;
t130 = t56.*9.296e-5;
t133 = t75.*9.296e-5;
t134 = t55.*9.485e-5;
t135 = t47.*7.962500000000001e-5;
t138 = t79.*9.485e-5;
t139 = t67.*7.962500000000001e-5;
t144 = -t141;
t172 = -t159;
t174 = -t162;
t183 = -t168;
t188 = -t173;
t199 = -t195;
t205 = -t201;
t227 = t5.*t224;
t228 = t11.*t224;
t229 = t63.*4.63864974683e-6;
t231 = t47.*4.002781743233e-5;
t232 = t70.*4.63864974683e-6;
t237 = t48.*3.52200536814e-6;
t239 = t48.*1.258507593186e-5;
t241 = -t238;
t243 = t67.*3.85924222008233e-3;
t244 = t69.*3.52200536814e-6;
t248 = t69.*1.258507593186e-5;
t251 = t62.*2.911421944783775e-4;
t253 = t68.*2.911421944783775e-4;
t299 = t180+t181+t193+t194+t298;
t301 = t126+t131+t158+t161+t186+t200+t226+t255+3.08503415834179e-2;
t303 = t99+t126+t131+t140+t148+t151+t155+t157+t164+t179+t182+t185+t192+t196+t206+t207+t226+t255+3.379819209690679e-1;
t94 = t39+t87;
t95 = t40+t86;
t96 = t7.*t92;
t98 = t13.*t92;
t104 = t55+t90;
t113 = -t111;
t142 = -t138;
t143 = -t139;
t145 = t109+t110;
t204 = t108+t119;
t208 = t7.*t12.*t97.*9.296e-5;
t209 = t112+t118;
t210 = t12.*t42.*t91.*1.5925e-4;
t215 = -t9.*(t109-t118);
t233 = -t229;
t235 = -t231;
t236 = -t232;
t242 = t130+t133;
t246 = -t243;
t247 = -t244;
t254 = -t251;
t264 = t136+t228;
t272 = t137+t227+2.37e+2./1.0e+3;
t302 = t148+t155+t164+t179+t182+t192+t206+t207+t301;
t103 = t7.*t94;
t105 = t13.*t94;
t114 = t74+t98;
t116 = t88+t96;
t156 = t108+t113;
t160 = t9.*t145;
t211 = t3.*t204;
t212 = t9.*t204;
t213 = t12.*t42.*t95.*1.5925e-4;
t217 = t12.*t13.*t104.*9.485e-5;
t219 = t209+3.3e+1./1.25e+2;
t249 = t134+t142;
t250 = t135+t143;
t257 = -t242.*(t77-t96);
t259 = t242.*(t77-t96);
t267 = t4.*t264;
t268 = t10.*t264;
t273 = t4.*t272;
t274 = t10.*t272;
t117 = t81+t103;
t120 = t89+t105;
t189 = t3.*t156;
t191 = -t160;
t216 = -t212;
t218 = -t217;
t220 = t3.*t219;
t221 = t9.*t219;
t261 = t114.*t249;
t262 = t211+t215;
t263 = -t249.*(t78-t105);
t269 = -t268;
t278 = t267+t274;
t256 = t189+t191;
t258 = t117.*t242;
t265 = t211+t221;
t266 = t216+t220;
t270 = -t2.*(t212-t220);
t271 = -t8.*(t212-t220);
t280 = t9.*t278;
t281 = t8.*(t102+t2.*(t212-t220)).*(t160-t189).*(2.2e+1./1.25e+2);
t283 = t269+t273+3.3e+1./1.25e+2;
t287 = t8.*t262.*(t102+t2.*(t212-t220)).*(-2.2e+1./1.25e+2);
t288 = t8.*t262.*(t102+t2.*(t212-t220)).*(2.2e+1./1.25e+2);
t292 = t213+t259+t261;
t260 = -t258;
t275 = t101+t271;
t276 = t107+t270;
t282 = -t281;
t284 = t3.*t283;
t290 = t8.*t265.*(t102+t2.*(t212-t220)).*(-2.2e+1./1.25e+2);
t291 = t8.*t265.*(t102+t2.*(t212-t220)).*(2.2e+1./1.25e+2);
t294 = t8.*t292;
t296 = -t2.*(-t210+t258+t249.*(t78-t105));
t297 = t2.*(-t210+t258+t249.*(t78-t105));
t279 = t2.*t275.*(t160-t189).*(-2.2e+1./1.25e+2);
t285 = -t284;
t286 = t2.*t262.*t275.*(2.2e+1./1.25e+2);
t289 = t2.*t265.*t275.*(2.2e+1./1.25e+2);
t293 = t210+t260+t263;
t295 = -t294;
t300 = t280+t285;
M = reshape([t4.*(-1.63367952e-2)+t11.*8.4990968397e-3+t140+t148+t155+t158+cos(t17).*2.536047323340805e-1-cos(t45).*1.63367952e-2-cos(t46).*3.99274128e-5+cos(t50).*9.9389672074375e-2-cos(t57).*3.58439274e-5-cos(t82).*5.82284388956755e-4-sin(t17).*1.61248862826e-4+sin(t45).*2.65188e-5+sin(t46).*9.4673483784e-3+sin(t50).*2.88759272e-5+sin(t57).*8.4990968397e-3-sin(t82).*9.27729949366e-6+t12.^2.*t42.^2.*1.5925e-4+t97.*t242+t104.*t249+(t2.*t240+t8.*t300).^2.*1.707+(t8.*t240-t2.*t300).^2.*1.707+t37.*(t37.*1.975e-3+t6.*t42.*7.8e-6-t12.*t42.*9.92e-5)+(t102+t2.*(t212-t220)).^2.*(2.2e+1./1.25e+2)+t275.^2.*(2.2e+1./1.25e+2)+t12.*t42.*(t37.*(-9.92e-5)+t6.*t42.*6.1e-6+t12.*t42.*1.6808e-3)+t6.*t42.*(t37.*7.8e-6+t6.*t42.*2.092e-3+t12.*t42.*6.1e-6)+4.762913488144671e-1,t144+t149+t153+t168+t172+t174+t188+t198+t199+t205+t208+t214+t218+t222+t225+t233+t235+t236+t237+t241+t245+t246+t248+t253+t254+t289+t291,t144+t168+t174+t198+t199+t205+t208+t214+t218+t233+t235+t236+t237+t241+t245+t246+t248+t253+t254+t286+t288,t144+t208+t218+t233+t235+t236+t237+t241+t245+t246+t248+t253+t254+t279+t282,t37.*(-2.72839557767695e-3)+t47.*3.85924222008233e-3-t67.*4.002781743233e-5+t147+t154+t162+t172+t183+t188+t199+t205+t239+t247-t13.*t97.*9.296e-5-t7.*t104.*9.485e-5+(t39.*(3.9e+1./4.0e+2)-t73.*(3.9e+1./4.0e+2)).*(t102+t2.*(t212-t220)).*(2.2e+1./1.25e+2)-t275.*(t44.*(3.9e+1./4.0e+2)+t71.*(3.9e+1./4.0e+2)).*(2.2e+1./1.25e+2),t250,t149+t153+t168+t172+t174+t188+t198+t199+t205+t214+t222+t225+t233+t235+t236+t237+t241+t245+t246+t248+t253+t254+t289+t291+t295+t297,t4.*2.029574976e-1+t10.*5.30376e-5-t27.*7.98548256e-5+t32.*1.89346967568e-2+t126+t131+t151+t157+t185+t196+t226+t255-t4.*t11.*1.110870341856e-1-t5.*t10.*1.110870341856e-1+t4.*t5.*t6.*7.98548256e-5-t4.*t5.*t12.*9.874216756800001e-3-t6.*t10.*t11.*7.98548256e-5+t10.*t11.*t12.*9.874216756800001e-3+9.851289596233629e-1,t303,t302,t299,t125,t168+t174+t198+t199+t205+t214+t233+t235+t236+t237+t241+t245+t246+t248+t253+t254+t286+t288+t295+t297,t303,t126+t131+t151+t157+t185+t196+t226+t255+3.379819209690679e-1,t301,t298,t125,t233+t235+t236+t237+t241+t245+t246+t248+t253+t254+t279+t282+t295+t297,t302,t301,t126+t131+t226+t255+3.08503415834179e-2,t277,t125,t31.*2.4685541892e-3-t37.*4.49540057767695e-3+t43.*2.21608841985e-3+t47.*1.96735222008233e-3-t53.*2.4685541892e-3-t61.*2.21608841985e-3+t67.*2.432218256767e-5+t154+t183+t188+t205+t239+t247-cos(t21+t28).*4.724999999999993e-7-cos(t21+t41).*2.362499999999996e-7-cos(t28+t35).*4.724999999999993e-7+cos(t35+t41).*2.362499999999996e-7-cos(t21+t59).*2.362499999999996e-7+cos(t35+t59).*2.362499999999996e-7,t299,t298,t277,cos(t21).*9.449999999999986e-7+4.49540057767695e-3,0.0,t250,t125,t125,t125,0.0,1.5925e-4],[6,6]);

== matlab function impendent_control/impedent_control1/MATLAB Function2 ==
  data: JaDown3 input; dX output; dq input
function dX = fcn(JaDown3,dq)
dX=JaDown3*dq;
end

== matlab function impendent_control/impedent_control1/MATLAB Function3 ==
  data: dX input; dx output; Pdot input
function dx = fcn(dX,Pdot)
dx=[Pdot;dX];
end

== matlab function impendent_control/impedent_control1/MATLAB Function4 ==
  data: JaDown3 input; Jana output; J input
function Jana = fcn(JaDown3,J)
Jana=[J(1:3,:);JaDown3];
end

== matlab function impendent_control/impedent_control1/MATLAB Function5 ==
  data: Jana input; dx output; dq input
function dx = fcn(Jana,dq)
dx=Jana*dq;
end
